simulink model "HW4"  (R2020a)
settings: Solver=ode1  StartTime=0.0  StopTime=10  FixedStep=0.01  RelTol=1e-3  EnableMultiTasking=on
libraries: arduinolib x2, THLlib x1
settings Model: SILPILModeSetting=veronly  ExtModeTrigDuration=2  Creator=da_co  LastModifiedBy=da_co
settings OptimizationCC: EnhancedBackFolding=on  PassReuseOutputArgsAs=Individual arguments  ZeroExternalMemoryAtStartup=off  ZeroInternalMemoryAtStartup=off  MaxStackSize=64  OptimizeBlockOrder=speed  DifferentSizesBufferReuse=on  OptimizationCustomize=off  EfficientTunableParamExpr=on
settings DebuggingCC: ParameterTunabilityLossMsg=error
settings HardwareCC: ProdBitPerInt=16  ProdBitPerPointer=16  ProdBitPerSizeT=16  ProdBitPerPtrDiffT=16  ProdLargestAtomicFloat=None  ProdWordSize=8  ProdHWDeviceType=Atmel->AVR  UseSimulinkCoderFeatures=off
settings SFSimCC: MATLABDynamicMemAlloc=off
settings RTWCC: SystemTargetFile=ert.tlc  HardwareBoard=Arduino Mega 2560  TLCOptions=-aInlineSetEventsForThisBaseRateFcn=TLC_FALSE -aSuppressMultiTaskScheduler=TLC_FALSE -aRateBasedStepFcn=1  TemplateMakefile=ert_default_tmf  RTWVerbose=off  Toolchain=Arduino AVR  BuildConfiguration=Faster Runs
settings CodeAppCC: ForceParamTrailComments=on  OperatorAnnotations=on  SimulinkDataObjDesc=on  SFDataObjDesc=on  MangleLength=10  InsertBlockDesc=on
settings ERTTargetCC: SupportContinuousTime=on  SupportVariableSizeSignals=on  ExtMode=on  ExtModeStaticAllocSize=2048  ExtModeMexArgs='127.0.0.1' 0 17725  ERTSrcFileBannerTemplate=codertarget_code_template.cgt  ERTHdrFileBannerTemplate=codertarget_code_template.cgt  ERTDataSrcFileTemplate=codertarget_code_template.cgt  ERTDataHdrFileTemplate=codertarget_code_template.cgt

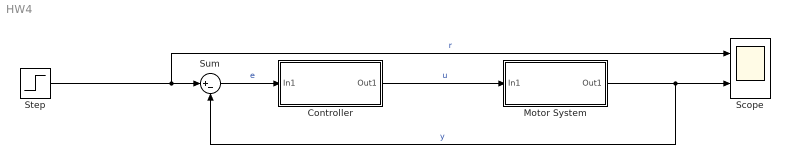
== system HW4 ==
  Controller : Subsystem
  Motor System : Subsystem
  Scope : Scope  NumInputPorts=2
  Step : Step  SampleTime=0
  Sum : Sum  Inputs=|+-
  wires:
  Controller/1(Out1) -> Motor System/1(In1)  "u"
  Motor System/1(Out1) -> Scope/2, Sum/2  "y"
  Sum/1 -> Controller/1(In1)  "e"
  Step/1 -> Scope/1, Sum/1  "r"

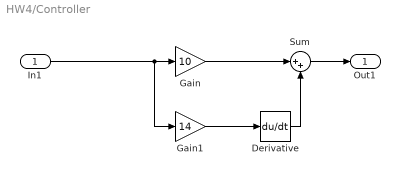
== system HW4/Controller ==
  In1 : Inport
  Derivative : Derivative
  Gain : Gain  Gain=10
  Gain1 : Gain  Gain=14
  Sum : Sum  Inputs=|++
  Out1 : Outport
  wires:
  In1/1 -> Gain1/1, Gain/1
  Sum/1 -> Out1/1
  Gain/1 -> Sum/1
  Derivative/1 -> Sum/2
  Gain1/1 -> Derivative/1

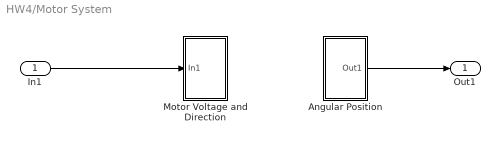
== system HW4/Motor System ==
  In1 : Inport
  Angular Position : Subsystem
  Motor Voltage and Direction : Subsystem
  Out1 : Outport
  wires:
  In1/1 -> Motor Voltage and Direction/1(In1)
  Angular Position/1(Out1) -> Out1/1

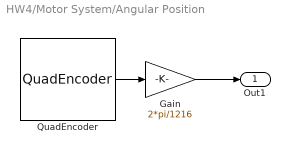
== system HW4/Motor System/Angular Position ==
  Gain : Gain  Gain=2*pi/1216
  QuadEncoder : THLlib/QuadEncoder  SystemSampleTime=-1  Latency=0  AutoFrameSizeCalculation=off
      settings: SourceProductName=Take Home Labs Arduino Support Package
  Out1 : Outport
  wires:
  QuadEncoder/1 -> Gain/1
  Gain/1 -> Out1/1

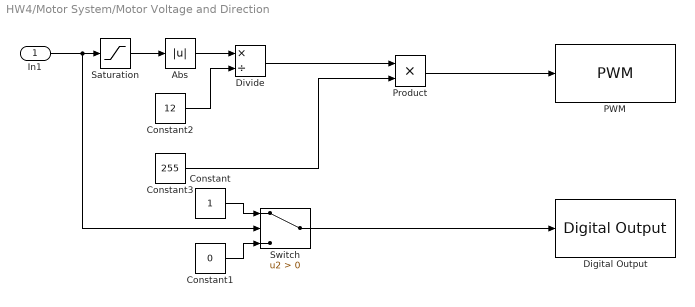
== system HW4/Motor System/Motor Voltage and Direction ==
  In1 : Inport
  Abs : Abs
  Constant : Constant
  Constant1 : Constant  Value=0
  Constant2 : Constant  Value=12
  Constant3 : Constant  Value=255
  Digital Output : arduinolib/Digital Output  pinNumber=4  Direction=output  blockPlatform=arduino
  Divide : Product  Inputs=*/
  PWM : arduinolib/PWM  pinNumber=5  frequencyType=Default  desiredFrequency=490.2  achievableFrequency=490.2
  Product : Product
  Saturation : Saturate  UpperLimit=12  LowerLimit=-12
  Switch : Switch  Criteria=u2 > Threshold
  wires:
  Constant2/1 -> Divide/2
  Divide/1 -> Product/1
  In1/1 -> Saturation/1, Switch/2
  Switch/1 -> Digital Output/1
  Abs/1 -> Divide/1
  Constant/1 -> Switch/1
  Product/1 -> PWM/1
  Constant3/1 -> Product/2
  Saturation/1 -> Abs/1
  Constant1/1 -> Switch/3
